simulink model "Driveline_ctrl_sim"  (R2020a)
settings: Solver=ode45  StartTime=0.0  StopTime=3  MaxStep=0.001  RelTol=1e-3
values from neighbouring files (symbols this model uses):
  A = [-ds/(Jf*i^2)  ds/(Jf*i) -cs/(Jf*i) ... (first row only)    [Driveline_ctrl_design.m]
  B = [1/Jf;0;0]    [Driveline_ctrl_design.m]
  B1 = [B H]    [Driveline_ctrl_design.m]
  C = eye(3)    [Driveline_ctrl_design.m]
  D = zeros(3,2)    [Driveline_ctrl_design.m]
  K = 1.0e+04*[0.0037    0.1915    1.3148]    [Driveline_ctrl_design.m]
  kr = 4.0033e+03    (= 4003.3)    [Driveline_ctrl_design.m]
  L = [l1 l2 l3]'    [Driveline_ctrl_design.m]
  x0 = [120 2 0]'    [Driveline_ctrl_design.m]
settings Model: Creator=jofr  LastModifiedBy=Tomas
settings DataIOCC: LimitDataPoints=on  SaveFormat=Array  SignalLoggingSaveFormat=ModelDataLogs  ReturnWorkspaceOutputs=off
settings OptimizationCC: BlockReduction=off  BooleanDataType=off  LifeSpan=inf
settings DebuggingCC: SaveWithParameterizedLinksMsg=none  UnderspecifiedInitializationDetection=Classic  MergeDetectMultiDrivingBlocksExec=none  SignalResolutionControl=TryResolveAllWithWarning  MultiTaskDSMMsg=warning  MultiTaskCondExecSysMsg=none  SFUnexpectedBacktrackingDiag=warning  SFNoUnconditionalDefaultTransitionDiag=warning  SFExecutionAtInitializationDiag=none  ArithmeticOperatorsInVariantConditions=warning
settings HardwareCC: ProdBitPerPointer=32  ProdBitPerSizeT=32  ProdBitPerPtrDiffT=32  ProdLargestAtomicFloat=None  ProdIntDivRoundTo=Undefined  ProdEndianess=Unspecified  ProdWordSize=32  ProdHWDeviceType=32-bit Generic  TargetUnknown=on
settings ModelReferenceCC: PropagateSignalLabelsOutOfModel=off
settings SFSimCC: SimUseLocalCustomCode=off  CustomCodeUndefinedFunction=UseInterfaceOnly
settings RTWCC: RTWUseLocalCustomCode=off
settings CodeAppCC: StateflowObjectComments=on
settings GRTTargetCC: TargetLangStandard=C89/C90 (ANSI)
settings ConfigComp: CovMetricSettings=dw  CovHtmlReporting=on  CovSaveCumulativeToWorkspaceVar=on  CovSaveSingleToWorkspaceVar=on  CovExternalEMLEnable=off

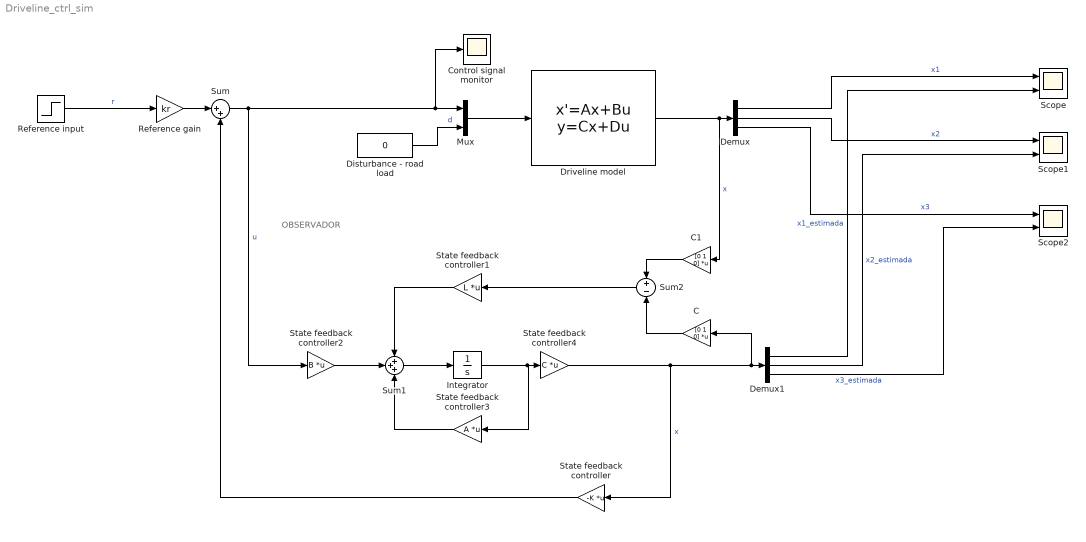
== system Driveline_ctrl_sim ==
  note: OBSERVADOR
  C : Gain  Gain=[0 1 0]  Multiplication=Matrix(K*u)
  C1 : Gain  Gain=[0 1 0]  Multiplication=Matrix(K*u)
  Control signal monitor : Scope
  Demux : Demux  Outputs=3
  Demux1 : Demux  Outputs=3
  Disturbance - road load : Constant  Value=0
  Driveline model : StateSpace  A=A  B=B1  C=C  D=D  InitialCondition=x0
  Integrator : Integrator
  Mux : Mux  Inputs=2
  Reference gain : Gain  Gain=kr
  Reference input : Step  Before=2  After=4  SampleTime=0
  Scope : Scope  NumInputPorts=2
  Scope1 : Scope  NumInputPorts=2
  Scope2 : Scope  NumInputPorts=2
  State feedback controller : Gain  Gain=-K  Multiplication=Matrix(K*u)
  State feedback controller1 : Gain  Gain=L  Multiplication=Matrix(K*u)
  State feedback controller2 : Gain  Gain=B  Multiplication=Matrix(K*u)
  State feedback controller3 : Gain  Gain=A  Multiplication=Matrix(K*u)
  State feedback controller4 : Gain  Gain=C  Multiplication=Matrix(K*u)
  Sum : Sum  Inputs=|++
  Sum1 : Sum  Inputs=+++
  Sum2 : Sum  Inputs=+|-
  wires:
  Driveline model/1 -> C1/1, Demux/1  "x"
  Demux/1 -> Scope/1  "x1"
  Demux/2 -> Scope1/1  "x2"
  Demux/3 -> Scope2/1  "x3"
  Mux/1 -> Driveline model/1
  Disturbance - road load/1 -> Mux/2  "d"
  State feedback controller/1 -> Sum/2
  Reference input/1 -> Reference gain/1  "r"
  Sum/1 -> Control signal monitor/1, Mux/1, State feedback controller2/1  "u"
  Reference gain/1 -> Sum/1
  State feedback controller4/1 -> C/1, Demux1/1, State feedback controller/1  "x"
  Demux1/3 -> Scope2/2  "x3_estimada"
  Demux1/1 -> Scope/2  "x1_estimada"
  Demux1/2 -> Scope1/2  "x2_estimada"
  C1/1 -> Sum2/1
  C/1 -> Sum2/2
  Sum2/1 -> State feedback controller1/1
  State feedback controller2/1 -> Sum1/2
  State feedback controller1/1 -> Sum1/1
  Sum1/1 -> Integrator/1
  State feedback controller3/1 -> Sum1/3
  Integrator/1 -> State feedback controller3/1, State feedback controller4/1
